simulink model "task4B_d"  (R2024b)
settings: Solver=VariableStepAuto  StartTime=0.0  StopTime=8000  RelTol=1e-3
settings Model: NumberOfSteps=100  Creator=brope  LastModifiedBy=brope

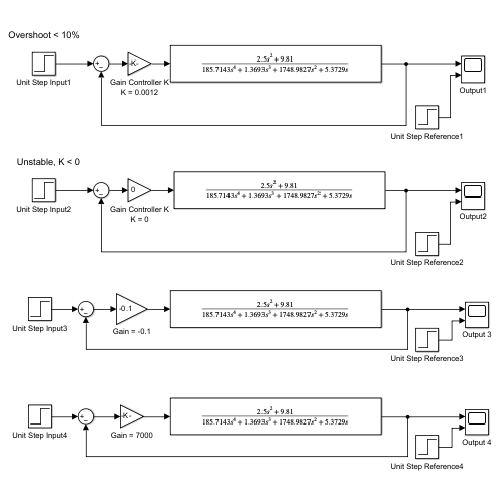
[thumbnail: Simulink's stored preview of the top-level diagram]
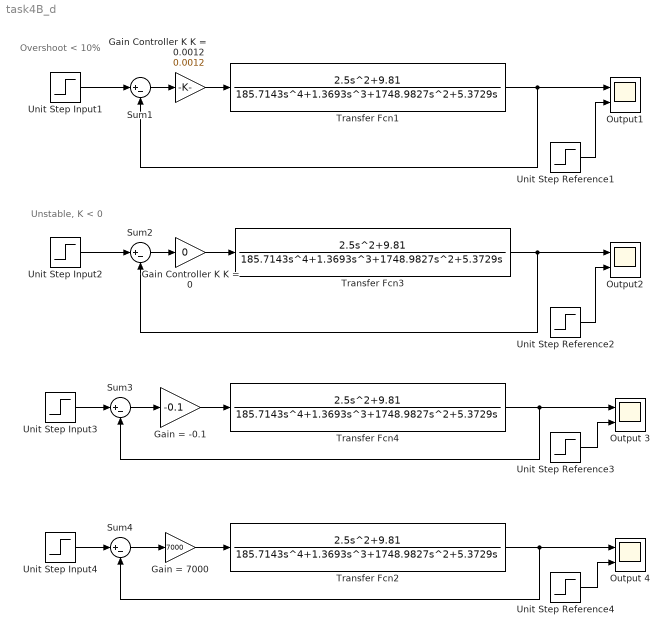
== system task4B_d ==
  note: Unstable, K < 0
  note: Overshoot < 10%
  Gain = -0.1 : Gain  Gain=-0.1
  Gain = 7000 : Gain  Gain=7000
  Gain Controller K K = 0 : Gain  Gain=0
  Gain Controller K K = 0.0012 : Gain  Gain=0.0012
  Output 3 : Scope  NumInputPorts=2
  Output 4 : Scope  NumInputPorts=2
  Output1 : Scope  NumInputPorts=2
  Output2 : Scope  NumInputPorts=2
  Sum{1..4} (4 alike) : Sum  Inputs=|+-
  Transfer Fcn{1..4} (4 alike) : TransferFcn  Numerator=[2.5 0 9.81]  Denominator=[185.7143 1.3693 1748.9827 5.3729 0]  ParameterTunability=Optimized
  Unit Step Input{1..4} (4 alike) : Step  SampleTime=0
  Unit Step Reference{1..4} (4 alike) : Step  SampleTime=0
  wires:
  Unit Step Input2/1 -> Sum2/1
  Unit Step Reference2/1 -> Output2/2
  Gain Controller K K = 0/1 -> Transfer Fcn3/1
  Gain Controller K K = 0.0012/1 -> Transfer Fcn1/1
  Unit Step Reference1/1 -> Output1/2
  Unit Step Input1/1 -> Sum1/1
  Gain = -0.1/1 -> Transfer Fcn4/1
  Sum3/1 -> Gain = -0.1/1
  Unit Step Input3/1 -> Sum3/1
  Transfer Fcn4/1 -> Sum3/2, Output 3/1
  Unit Step Reference3/1 -> Output 3/2
  Unit Step Input4/1 -> Sum4/1
  Transfer Fcn2/1 -> Sum4/2, Output 4/1
  Unit Step Reference4/1 -> Output 4/2
  Sum4/1 -> Gain = 7000/1
  Gain = 7000/1 -> Transfer Fcn2/1
  Sum1/1 -> Gain Controller K K = 0.0012/1
  Transfer Fcn1/1 -> Output1/1, Sum1/2
  Sum2/1 -> Gain Controller K K = 0/1
  Transfer Fcn3/1 -> Output2/1, Sum2/2
